simulink model "LTI"  (R2020a)
settings: Solver=VariableStepAuto  StartTime=0.0  StopTime=100  RelTol=1e-3
libraries: cstblocks x1
settings Model: Creator=WASHINGTON  LastModifiedBy=WASHINGTON

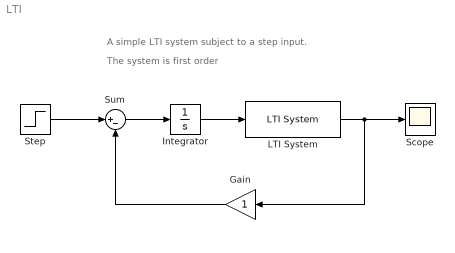
== system LTI ==
  note: The system is first order
  note: A simple LTI system subject to a step input.
  Gain : Gain
  Integrator : Integrator
  LTI System : cstblocks/LTI System  sys=tf(1,[4 4])  IC=[]
  Scope : Scope
  Step : Step  SampleTime=0
  Sum : Sum  Inputs=|+-
  wires:
  Integrator/1 -> LTI System/1
  Sum/1 -> Integrator/1
  Gain/1 -> Sum/2
  LTI System/1 -> Scope/1, Gain/1
  Step/1 -> Sum/1
